simulink model "EMGRecorder"  (R2019a)
settings: Solver=VariableStepAuto  StartTime=0.0  StopTime=inf  RelTol=1e-3
undefined symbols (not defined in the file or in its folder): daq
libraries: daqlib x1, arduinolib x1, simulink x1
settings Model: Creator=Kusunoki  LastModifiedBy=Kusunoki

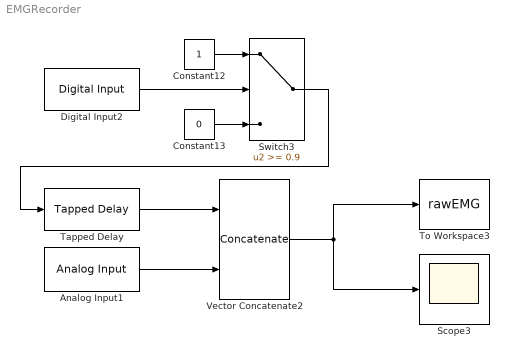
== system EMGRecorder ==
  Analog Input1 : daqlib/Analog Input  DeviceMenu=(none)  Device=ni Dev1 (USB-6000)  ObjConstructor=daq.createSession('ni')  NChannelsSelected=1  Channels=1$ai0$$Dev1$1$1$1$1$#0$ai1$$Dev1$1$1$1$1$#0$ai2$$Dev1$1$1$1$1$#0$ai3$$Dev1$1$1$1$1$#0$ai4$$Dev1$1$1$1$1$#0$ai5$$Dev1$1$1$1$1$#0$ai6$$Dev1$1$1$1$1$#0$ai7$$Dev1$1$1$1$1$#  NPorts=1 per channel  SampleRate=2000  ActualRate=2000  ScansPerTrigger=200  OutputTimestamp=off  AcqMode=0  NumFrameBuffer=100  OutputTriggertime=off
      settings: SourceProductName=Data Acquisition Toolbox  SourceProductBaseCode=DA
  Constant12 : Constant
  Constant13 : Constant  Value=0
  Digital Input2 : arduinolib/Digital Input  pinNumber=8  sampleTime=0.0005  blockPlatform=arduino
      settings: SourceProductName=Simulink Support Package for Arduino Hardware
  Scope3 : Scope
  Switch3 : Switch  Threshold=0.9
  Tapped Delay : simulink/Discrete/Tapped Delay  vinit=0.0  samptime=-1  NumDelays=200  DelayOrder=Oldest  includeCurrent=off
  To Workspace3 : ToWorkspace  VariableName=rawEMG  SaveFormat=Timeseries  SampleTime=-1
  Vector Concatenate2 : Concatenate  Mode=Multidimensional array  ConcatenateDimension=2
  wires:
  Constant12/1 -> Switch3/1
  Digital Input2/1 -> Switch3/2
  Constant13/1 -> Switch3/3
  Analog Input1/1 -> Vector Concatenate2/2
  Vector Concatenate2/1 -> To Workspace3/1, Scope3/1
  Tapped Delay/1 -> Vector Concatenate2/1
  Switch3/1 -> Tapped Delay/1
